simulink model "Current_reversible_chopper"  (Simulink 6.1)
settings: Solver=ode23tb  StartTime=0.0  StopTime=0.03  MaxStep=2e-5  RelTol=1e-3  AbsTol=.1
libraries: powerlib x7
settings Model: LastModifiedBy=ThinkPad
settings DebuggingCC: SolverPrmCheckMsg=warning

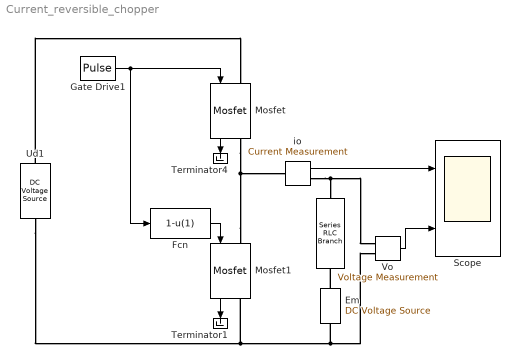
== system Current_reversible_chopper ==
  " " : powerlib/Elements/Series RLC Branch  Orientation=down  PhysicalDomain=powersysdomain  SubClassName=unknown  LeftPortType=p1  RightPortType=p1  LConnTagsString=__new0  RConnTagsString=__new0  Resistance=1  Inductance=0.001  Capacitance=inf  Measurements=None
  Em : powerlib/Electrical Sources/DC Voltage Source  Orientation=up  Amplitude=50  Measurements=None
  Fcn : Fcn  Expr=1-u(1)
  Gate Drive1 : DiscretePulseGenerator  PulseType=Time based  Period=0.001  PulseWidth=70
  Mosfet : powerlib/Power Electronics/Mosfet  Orientation=down  Ron=0.001  Lon=1e-9  Rd=.001  IC=0  Rs=1  Cs=1e-6  Measurements=on
  Mosfet1 : powerlib/Power Electronics/Mosfet  Orientation=down  Ron=0.001  Lon=1e-9  Rd=.001  IC=0  Rs=1  Cs=1e-6  Measurements=on
  Scope : Scope  NumInputPorts=2
      settings: TimeRange=0.01  YMin=-100~-50  YMax=100~150  SampleTime=2e-4
  Terminator1 : Terminator
      settings: Orientation=down
  Terminator4 : Terminator
      settings: Orientation=down
  Ud1 : powerlib/Electrical Sources/DC Voltage Source  Orientation=up  Amplitude=100  Measurements=None
  Vo : powerlib/Measurements/Voltage Measurement  PhasorSimulation=off  OutputType=Complex  PSBequivalent=0
  io : powerlib/Measurements/Current Measurement  PhasorSimulation=off  OutputType=Complex  PSBequivalent=0
  wires:
  Vo/1 -> Scope/2
  Fcn/1 -> Mosfet1/1
  Gate Drive1/1 -> Fcn/1, Mosfet/1
  io/1 -> Scope/1
  Mosfet/1 -> Terminator4/1
  Mosfet1/1 -> Terminator1/1
  connections:
  Mosfet1/RConn1 -- Em/LConn1 -- Vo/LConn2 -- Ud1/LConn1
  Mosfet1/LConn1 -- io/LConn1 -- Mosfet/RConn1
  Ud1/RConn1 -- Mosfet/LConn1
  io/RConn1 -- " "/LConn1 -- Vo/LConn1
  Em/RConn1 -- " "/RConn1
